simulink model "converter"  (R2018a)
settings: Solver=VariableStepAuto  StartTime=0.0  StopTime=10.0  RelTol=1e-3
settings Model: Creator=Edoardo Debenedetti  LastModifiedBy=Edoardo Debenedetti

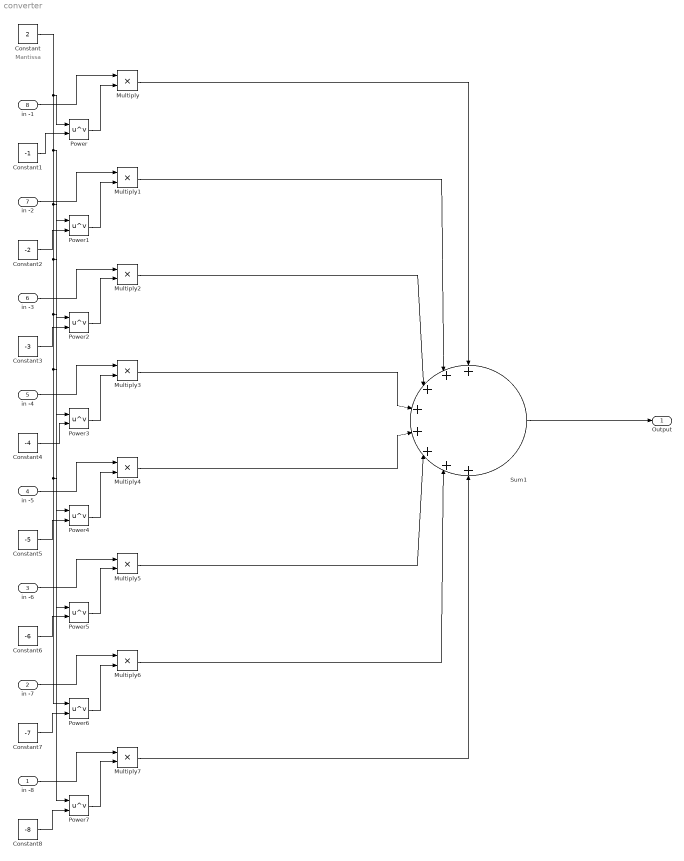
== system converter ==
  note: Mantissa
  in -8 : Inport  OutDataTypeStr=boolean
  in -7 : Inport  Port=2  OutDataTypeStr=boolean
  in -6 : Inport  Port=3  OutDataTypeStr=boolean
  in -5 : Inport  Port=4  OutDataTypeStr=boolean
  in -4 : Inport  Port=5  OutDataTypeStr=boolean
  in -3 : Inport  Port=6  OutDataTypeStr=boolean
  in -2 : Inport  Port=7  OutDataTypeStr=boolean
  in -1 : Inport  Port=8  OutDataTypeStr=boolean
  Constant : Constant  Value=2
  Constant1 : Constant  Value=-1
  Constant2 : Constant  Value=-2
  Constant3 : Constant  Value=-3
  Constant4 : Constant  Value=-4
  Constant5 : Constant  Value=-5
  Constant6 : Constant  Value=-6
  Constant7 : Constant  Value=-7
  Constant8 : Constant  Value=-8
  Multiply{,1..7} (8 alike) : Product
  Power{,1..7} (8 alike) : Math  Operator=pow  SaturateOnIntegerOverflow=on
  Sum1 : Sum  Inputs=8
  Output : Outport
  wires:
  Constant1/1 -> Power/2
  Power/1 -> Multiply/2
  in -1/1 -> Multiply/1
  in -2/1 -> Multiply1/1
  Power1/1 -> Multiply1/2
  Constant2/1 -> Power1/2
  Constant3/1 -> Power2/2
  Power2/1 -> Multiply2/2
  in -3/1 -> Multiply2/1
  in -5/1 -> Multiply4/1
  Power4/1 -> Multiply4/2
  Constant5/1 -> Power4/2
  Constant4/1 -> Power3/2
  Power3/1 -> Multiply3/2
  in -4/1 -> Multiply3/1
  in -8/1 -> Multiply7/1
  Power7/1 -> Multiply7/2
  Constant8/1 -> Power7/2
  in -7/1 -> Multiply6/1
  Power6/1 -> Multiply6/2
  Constant7/1 -> Power6/2
  Constant6/1 -> Power5/2
  Power5/1 -> Multiply5/2
  in -6/1 -> Multiply5/1
  Multiply/1 -> Sum1/1
  Multiply1/1 -> Sum1/2
  Multiply2/1 -> Sum1/3
  Multiply3/1 -> Sum1/4
  Multiply4/1 -> Sum1/5
  Multiply5/1 -> Sum1/6
  Multiply6/1 -> Sum1/7
  Multiply7/1 -> Sum1/8
  Sum1/1 -> Output/1
  Constant/1 -> Power3/1, Power5/1, Power6/1, Power7/1, Power4/1, Power2/1, Power1/1, Power/1
